simulink model "FM_Mod_Self_Module_Sine"  (R2018b)
settings: Solver=VariableStepAuto  StartTime=0.0  StopTime=2*10^-3  RelTol=1e-3
undefined symbols (not defined in the file or in its folder): DiscIntNeverNeededParam
settings Model: Creator=lenovo  LastModifiedBy=lenovo

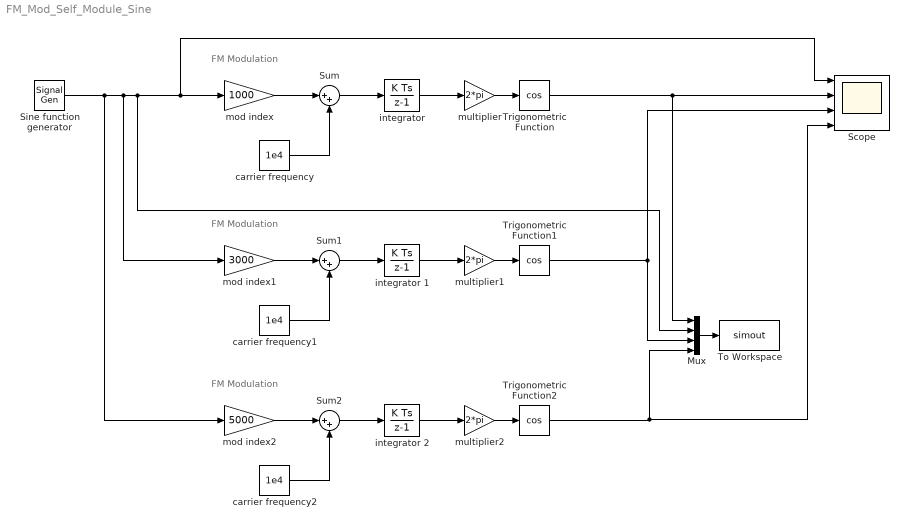
== system FM_Mod_Self_Module_Sine ==
  note: FM Modulation
  note: FM Modulation
  note: FM Modulation
  Mux : Mux
  Scope : Scope  NumInputPorts=4
  "Sine function generator " : SignalGenerator  Amplitude=1.5  Frequency=1e3
  Sum : Sum  Inputs=|++
  Sum1 : Sum  Inputs=|++
  Sum2 : Sum  Inputs=|++
  To Workspace : ToWorkspace  VariableName=simout  SaveFormat=Timeseries  SampleTime=-1
  Trigonometric Function : Trigonometry  Operator=cos
  Trigonometric Function1 : Trigonometry  Operator=cos
  Trigonometric Function2 : Trigonometry  Operator=cos
  carrier frequency : Constant  Value=1e4
  carrier frequency1 : Constant  Value=1e4
  carrier frequency2 : Constant  Value=1e4
  "integrator " : DiscreteIntegrator  SampleTime=1/1000000  ICPrevOutput=DiscIntNeverNeededParam  ICPrevScaledInput=DiscIntNeverNeededParam
  integrator 1 : DiscreteIntegrator  SampleTime=1/1000000  ICPrevOutput=DiscIntNeverNeededParam  ICPrevScaledInput=DiscIntNeverNeededParam
  integrator 2 : DiscreteIntegrator  SampleTime=1/1000000  ICPrevOutput=DiscIntNeverNeededParam  ICPrevScaledInput=DiscIntNeverNeededParam
  mod index : Gain  Gain=1000
  mod index1 : Gain  Gain=3000
  mod index2 : Gain  Gain=5000
  multiplier : Gain  Gain=2*pi
  multiplier1 : Gain  Gain=2*pi
  multiplier2 : Gain  Gain=2*pi
  wires:
  "Sine function generator "/1 -> mod index2/1, mod index1/1, Mux/2, mod index/1, Scope/1
  "integrator "/1 -> multiplier/1
  Mux/1 -> To Workspace/1
  carrier frequency/1 -> Sum/2
  Sum/1 -> "integrator "/1
  multiplier/1 -> Trigonometric Function/1
  mod index/1 -> Sum/1
  Trigonometric Function/1 -> Scope/2, Mux/1
  mod index1/1 -> Sum1/1
  multiplier1/1 -> Trigonometric Function1/1
  Sum1/1 -> integrator 1/1
  carrier frequency1/1 -> Sum1/2
  integrator 1/1 -> multiplier1/1
  integrator 2/1 -> multiplier2/1
  carrier frequency2/1 -> Sum2/2
  Sum2/1 -> integrator 2/1
  multiplier2/1 -> Trigonometric Function2/1
  mod index2/1 -> Sum2/1
  Trigonometric Function1/1 -> Mux/3, Scope/3
  Trigonometric Function2/1 -> Scope/4, Mux/4
